simulink model "Task1_idealSystem_runner"  (R2025b)
settings: Solver=VariableStepAuto  StartTime=0.0  StopTime=(3600+37*60/24)*24*7  RelTol=1e-3
libraries: fl_lib x14, nesl_utility x6, simulink x2, ee_lib x1
settings Model: Creator=gdudgeon  LastModifiedBy=stefano
settings RTWCC: GPUComputeCapability=3.5

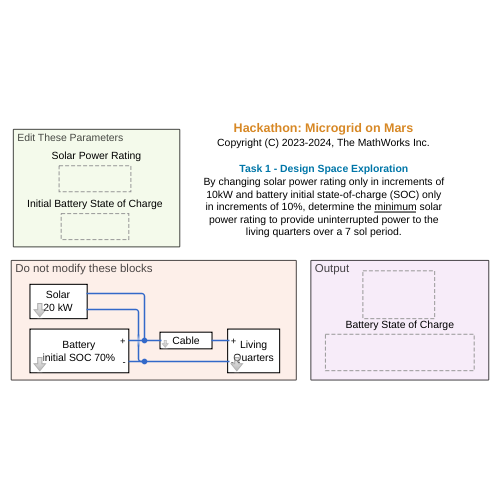
[thumbnail: Simulink's stored preview of the top-level diagram]
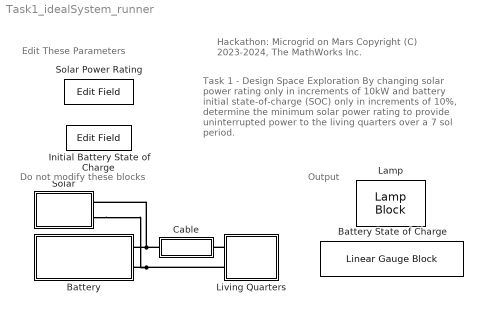
== system Task1_idealSystem_runner ==
  note: Task 1 - Design Space Exploration
      | By changing solar power rating only in increments of 10kW and battery initial state-of-charge (SOC) only in increments of 10%, determine the minimum solar power rating to provide uninterrupted power to the living quarters over a 7 sol period.
  note: Output
  note: Edit These Parameters
  note: Do not modify these blocks
  note: Hackathon: Microgrid on Mars
      | Copyright (C) 2023-2024, The MathWorks Inc.
  " Solar Power Rating" : EditField  Tag=Solar kW  Description=Solar kW  LabelPosition=Hide  ShowInitialText=on  Alignment=Center
  Battery : Subsystem  mask{initSOC=70}
      mask prompts: initSOC "Initial SOC (%)"
      mask Display:
      | isoc = get(gcbh,'initSOC');
      | 
      | disp(['Battery\ninitial SOC ',isoc,'%'])
  Battery State of Charge : LinearGaugeBlock  LabelPosition=Hide  FontColor=[0.0, 0.0, 0.0]
  Cable : Subsystem
      mask Display: disp('Cable')
  Initial Battery State of Charge : EditField  LabelPosition=Hide  ShowInitialText=on  Alignment=Center
  Lamp : LampBlock  DefaultColor=[255.0, 0.0, 0.0]
  Living Quarters : Subsystem
      mask Display: disp('Living\nQuarters')
  Solar : Subsystem  mask{power_rating=20}
      mask prompts: power_rating "Power Rating (kW)"
      mask Display:
      | pr = get(gcbh,'power_rating');
      | disp(['Solar\n',pr,' kW'])
  connections:
  Solar/RConn2 -- Living Quarters/LConn2 -- Battery/RConn2
  Cable/LConn1 -- Solar/RConn1 -- Battery/RConn1
  Living Quarters/LConn1 -- Cable/RConn1

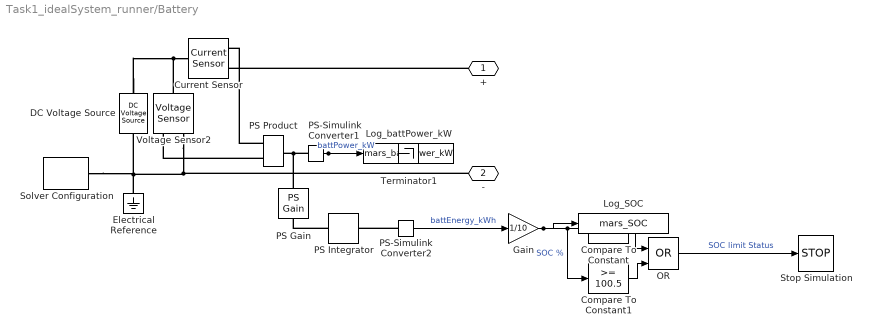
== system Task1_idealSystem_runner/Battery ==
  Compare To Constant : simulink/Logic and Bit Operations/Compare To Constant  relop=<=  const=0  OutDataTypeStr=boolean
  Compare To Constant1 : simulink/Logic and Bit Operations/Compare To Constant  relop=>=  const=100.5  OutDataTypeStr=boolean
  Current Sensor : fl_lib/Electrical/Electrical Sensors/Current Sensor
  DC Voltage Source : fl_lib/Electrical/Electrical Sources/DC Voltage Source  v0=510 V
  Electrical Reference : fl_lib/Electrical/Electrical Elements/Electrical Reference
  Gain : Gain  Gain=1/10
  Log_SOC : ToWorkspace  VariableName=mars_SOC  SaveFormat=Structure With Time  SampleTime=-1
  Log_battPower_kW : ToWorkspace  VariableName=mars_battPower_kW  SaveFormat=Structure With Time  SampleTime=-1
  OR : Logic  Operator=OR  IconShape=distinctive  AllPortsSameDT=off  OutDataTypeStr=boolean
  PS Gain : fl_lib/Physical Signals/Functions/PS Gain  gain=-1
  PS Integrator : fl_lib/Physical Signals/Linear Operators/PS Integrator  reset_method=foundation.enum.IntegratorResetSpec.None  initial_condition_spec=foundation.enum.IntegratorICSpec.Internal  saturation_spec=foundation.enum.IntegratorSaturationSpec.None  saturation_source_spec=foundation.enum.IntegratorSaturationSourceSpec.Internal  x0=initSOC*10 kW*hr  xu=inf s  xl=-inf s
  PS Product : fl_lib/Physical Signals/Functions/PS Product
  PS-Simulink Converter1 : nesl_utility/PS-Simulink Converter  PhysicalDomain=network_engine_domain  SubClassName=ps_output  LeftPortType=input  RightPortType=output  PseudoPeriodic=off  Frequencies=[]  VectorFormat=inherit  Unit=kW  AffineConversion=off
  PS-Simulink Converter2 : nesl_utility/PS-Simulink Converter  PhysicalDomain=network_engine_domain  SubClassName=ps_output  LeftPortType=input  RightPortType=output  PseudoPeriodic=off  Frequencies=[]  VectorFormat=inherit  Unit=kW*hr  AffineConversion=off
  Solver Configuration : nesl_utility/Solver Configuration  PhysicalDomain=network_engine_domain  SubClassName=solver  LeftPortType=input  RightPortType=generic  Tones=[]  Harmonics=[]  SimulateNoise=off  Profile=off  UseLocalSampling=off  EnableSwitchedLinearOptims=on  FrequencyDomain=off  UseCCode=off  RelTol=0.001  AbsTol=0.001  MinStep=1e-09  ToWorkspace=off  RevertToSquareIcSolve=off  NumHomotopyIterations=100  PhasorMode=off  PhasorModeNumHarmonics=1  ConsistencySolver=NEWTON_XTOL_AFTER_FTOL  IndexReductionMethod=DerivativeReplacement  DoDC=off  ResidualTolerance=1e-09  ConsistencyTolSource=GLOBAL  ConsistencyAbsTol=0.001  ConsistencyRelTol=0.001  ConsistencyTolFactor=0.001  UseLocalSolver=on  LocalSolverChoice=NE_BACKWARD_EULER_ADVANCER  ResolveIndetEquations=off  FunctionEvalNumThread=1  LocalSolverSampleTime=Ts  DoFixedCost=on  MaxNonlinIter=1  MaxModeIter=2  ComputeImpulses=off  ImpulseIterations=2  LinearAlgebra=auto  LinearAlgebraNumThread=0  EquationFormulation=NE_TIME_EF  DelaysMemoryBudget=1024  AutomaticFiltering=off  FilteringTimeConstant=0.001  PartitionStorageMethod=AS_NEEDED  PartitionMemoryBudget=1024  PartitionMethod=ROBUST  MultibodyUseLocalSolver=off  MultibodyLocalSolverChoice=ODE1  MultibodyLocalSolverSampleTime=0.001
  Stop Simulation : Stop
  Terminator1 : Terminator
  Voltage Sensor2 : fl_lib/Electrical/Electrical Sensors/Voltage Sensor
  + : PMIOPort  Side=Right
  - : PMIOPort  Port=2  Side=Right
  wires:
  Gain/1 -> Compare To Constant1/1, Compare To Constant/1, Log_SOC/1  "SOC %"
  PS-Simulink Converter2/1 -> Gain/1  "battEnergy_kWh"
  PS-Simulink Converter1/1 -> Terminator1/1, Log_battPower_kW/1  "battPower_kW"
  OR/1 -> Stop Simulation/1  "SOC limit Status"
  Compare To Constant/1 -> OR/1
  Compare To Constant1/1 -> OR/2
  connections:
  DC Voltage Source/LConn1 -- Current Sensor/LConn1 -- Voltage Sensor2/LConn1
  PS Product/LConn2 -- Voltage Sensor2/RConn1
  PS-Simulink Converter2/LConn1 -- PS Integrator/RConn1
  Voltage Sensor2/RConn2 -- Solver Configuration/RConn1 -- DC Voltage Source/RConn1 -- Electrical Reference/LConn1 -- -/RConn1
  PS Product/LConn1 -- Current Sensor/RConn1
  PS Gain/LConn1 -- PS Product/RConn1 -- PS-Simulink Converter1/LConn1
  PS Integrator/LConn1 -- PS Gain/RConn1
  +/RConn1 -- Current Sensor/RConn2

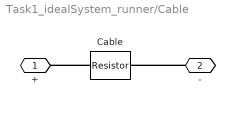
== system Task1_idealSystem_runner/Cable ==
  Cable : fl_lib/Electrical/Electrical Elements/Resistor  R=0.05 Ohm  i_specify=off  i_priority=None  i=0 A  i_nominal_specify=off  i_nominal_value=1  i_nominal_unit=A  v_specify=off  v_priority=None  v=0 V  v_nominal_specify=off  v_nominal_value=1  v_nominal_unit=V
  + : PMIOPort  Side=Left
  - : PMIOPort  Port=2  Side=Right
  connections:
  Cable/LConn1 -- +/RConn1
  -/RConn1 -- Cable/RConn1

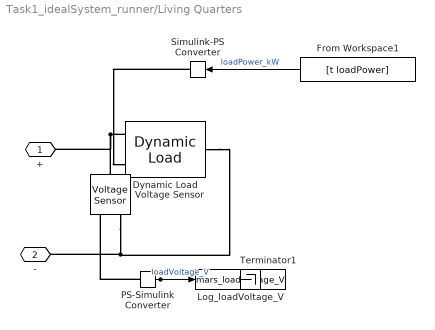
== system Task1_idealSystem_runner/Living Quarters ==
  Dynamic Load : ee_lib/Passive/Dynamic Load  load_type=ee.enum.dc_ac.dc  min_supply_voltage=20 V  pow_min=1e-3 W  G_reverse=1e-6 S  deltaV=1e-3 V  f0=60 Hz  Vrms_min=200 V  tau=0.01 s  Vrms_ini=300 V  Vang_ini=0 deg
      settings: InternalSimscapePortConfiguration="{\"Bottom\":[],\"Left\":[{\"id\":\"p\",\"label\":\"+\",\"type\":\"foundation.electrical.electrical\"}],\"Right\":[{\"id\":\"n\",\"label\":\"-\",\"type\":\"foundation.electrical.electrical\"}],\"Top\":[{\"id\":\"P\",\"label\":\"P\",\"type\":\"input\"}]}"
  From Workspace1 : FromWorkspace  VariableName=[t loadPower]
  Log_loadVoltage_V : ToWorkspace  VariableName=mars_loadVoltage_V  SaveFormat=Structure With Time  SampleTime=-1
  PS-Simulink Converter : nesl_utility/PS-Simulink Converter  PhysicalDomain=network_engine_domain  SubClassName=ps_output  LeftPortType=input  RightPortType=output  PseudoPeriodic=off  Frequencies=[]  VectorFormat=inherit  Unit=inherit  AffineConversion=off
  Simulink-PS Converter : nesl_utility/Simulink-PS Converter  PhysicalDomain=network_engine_domain  SubClassName=ps_input  LeftPortType=input  RightPortType=output  PseudoPeriodic=off  Frequencies=[]  NoiseDistribution=none  NoiseParameters=[]  Unit=kW  AffineConversion=off  FilteringAndDerivatives=provide  SimscapeFilterOrder=1  InputFilterTimeConstant=0.001  UdotUserProvided=0
  Terminator1 : Terminator
  Voltage Sensor : fl_lib/Electrical/Electrical Sensors/Voltage Sensor
  + : PMIOPort  Side=Left
  - : PMIOPort  Port=2  Side=Left
  wires:
  From Workspace1/1 -> Simulink-PS Converter/1  "loadPower_kW"
  PS-Simulink Converter/1 -> Terminator1/1, Log_loadVoltage_V/1  "loadVoltage_V"
  connections:
  Dynamic Load/RConn1 -- Voltage Sensor/RConn2 -- -/RConn1
  Dynamic Load/LConn1 -- +/RConn1 -- Voltage Sensor/LConn1
  PS-Simulink Converter/LConn1 -- Voltage Sensor/RConn1
  Simulink-PS Converter/RConn1 -- Dynamic Load/LConn2

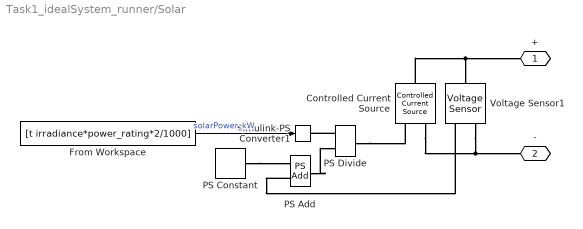
== system Task1_idealSystem_runner/Solar ==
  Controlled Current Source : fl_lib/Electrical/Electrical Sources/Controlled Current Source
  From Workspace : FromWorkspace  VariableName=[t irradiance*power_rating*2/1000]
  PS Add : fl_lib/Physical Signals/Functions/PS Add
  PS Constant : fl_lib/Physical Signals/Sources/PS Constant  constant=1e-6 V
  PS Divide : fl_lib/Physical Signals/Functions/PS Divide
  Simulink-PS Converter1 : nesl_utility/Simulink-PS Converter  PhysicalDomain=network_engine_domain  SubClassName=ps_input  LeftPortType=input  RightPortType=output  PseudoPeriodic=off  Frequencies=[]  NoiseDistribution=none  NoiseParameters=[]  Unit=kW  AffineConversion=off  FilteringAndDerivatives=provide  SimscapeFilterOrder=1  InputFilterTimeConstant=0.001  UdotUserProvided=0
  Voltage Sensor1 : fl_lib/Electrical/Electrical Sensors/Voltage Sensor
  + : PMIOPort  Side=Right
  - : PMIOPort  Port=2  Side=Right
  wires:
  From Workspace/1 -> Simulink-PS Converter1/1  "solarPower_kW"
  connections:
  PS Constant/RConn1 -- PS Add/LConn1
  Controlled Current Source/LConn1 -- Voltage Sensor1/LConn1 -- +/RConn1
  PS Divide/RConn1 -- Controlled Current Source/RConn1
  Voltage Sensor1/RConn2 -- Controlled Current Source/RConn2 -- -/RConn1
  PS Add/RConn1 -- PS Divide/LConn2
  PS Add/LConn2 -- Voltage Sensor1/RConn1
  PS Divide/LConn1 -- Simulink-PS Converter1/RConn1
